simulink model "Accelerometer"  (R2020b)
settings: Solver=FixedStepDiscrete  StartTime=0.0  StopTime=10.0  FixedStep=0.01  RelTol=1e-3  EnableMultiTasking=on
InitFcn:
  | mbd_s32k_consistency_checks(bdroot(gcs));
undefined symbols (not defined in the file): LQFP
libraries: mbd_s32k1xx_ec_toolbox x18, simulink x10
Description:
  | Sample code for extracting X,Y,Z components of acceleration from the on-board sensor.
  | 
  | Extra Modules (In addition to template defaults):
  | LPSPI0 (Accelerometer connection)
  | 
  | For more information, see our Accelerometer Guide:
  | https://www.audesseinc.com/labs/resources/accelerometer-guide/
  | 
  | Revision: 1.2
settings Model: LastModifiedBy=prasa
settings DataIOCC: ExternalInput=off  InitialState=off  SaveOutput=off  SignalLogging=off  SaveTime=off
settings OptimizationCC: DefaultParameterBehavior=Inlined  DefaultUnderspecifiedDataType=single  EnhancedBackFolding=on  PassReuseOutputArgsAs=Individual arguments  OptimizeBlockOrder=speed  EfficientTunableParamExpr=on
settings DebuggingCC: InheritedTsInSrcMsg=none  SingleTaskRateTransMsg=error  ParameterTunabilityLossMsg=error  UnconnectedInputMsg=error  UnconnectedOutputMsg=error  UnconnectedLineMsg=error  UnknownTsInhSupMsg=error  ArithmeticOperatorsInVariantConditions=warning
settings HardwareCC: ProdBitPerPointer=32  ProdBitPerSizeT=32  ProdBitPerPtrDiffT=32  ProdLargestAtomicInteger=Long  ProdLargestAtomicFloat=Double  ProdWordSize=32  ProdHWDeviceType=ARM Compatible->ARM Cortex
settings SFSimCC: MATLABDynamicMemAlloc=off  CustomCodeUndefinedFunction=UseInterfaceOnly
settings RTWCC: Description=Model Based Design Toolbox S32K1xx Code Generation Target  SystemTargetFile=mbd_s32k.tlc  MakeCommand=mbd_s32k_make_rtw COPY_MDLREF_INCLUDES=0  TemplateMakefile=mbd_s32k.tmf  GenerateReport=on  IncludeHyperlinkInReport=on  LaunchReport=on  GenerateTraceInfo=on  GenerateTraceReport=on  GenerateTraceReportSl=on  GenerateTraceReportSf=on  GenerateTraceReportEml=on
settings CodeAppCC: ForceParamTrailComments=on  IgnoreCustomStorageClasses=off  OperatorAnnotations=on  SimulinkDataObjDesc=on  SFDataObjDesc=on  InsertBlockDesc=on  StateflowObjectComments=on
settings STFCustomTargetCC: TargetLangStandard=C99 (ISO)  MultiwordLength=256  ConcurrentExecutionCompliant=off  CombineOutputUpdateFcns=on  ERTCustomFileBanners=on  SupportContinuousTime=off  SupportNonInlinedSFcns=off  RemoveResetFunc=on  MATLABClassNameForMDSCustomization=Simulink.SoftwareTarget.ERTCustomization  CPPClassGenCompliant=off  GRTInterface=off  SystemTargetFile=mbd_s32k.tlc
settings ERTTargetCC: TargetLangStandard=C99 (ISO)  ParMdlRefBuildCompliant=off  CompOptLevelCompliant=off  ConcurrentExecutionCompliant=off  ModelStepFunctionPrototypeControlCompliant=off  CPPClassGenCompliant=off  UseToolchainInfoCompliant=off  InlinedParameterPlacement=NonHierarchical  ERTSrcFileBannerTemplate=mbd_ert_code_template.cgt  ERTHdrFileBannerTemplate=mbd_ert_code_template.cgt  ERTDataSrcFileTemplate=mbd_ert_code_template.cgt  ERTDataHdrFileTemplate=mbd_ert_code_template.cgt  ERTCustomFileTemplate=example_file_process.tlc

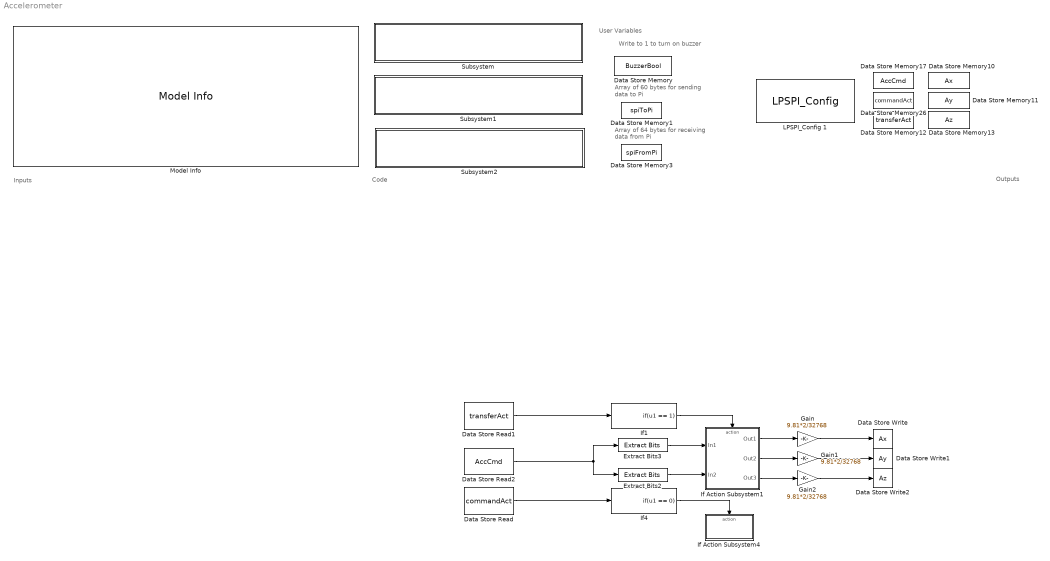
== system Accelerometer ==
  note: User Variables
  note: Write to 1 to turn on buzzer
  note: Array of 60 bytes for sending data to Pi
  note: Inputs
  note: Code
  note: Outputs
  note: Array of 64 bytes for receiving data from Pi
  Data Store Memory : DataStoreMemory  DataStoreName=BuzzerBool  ReadBeforeWriteMsg=warning  WriteAfterWriteMsg=warning  WriteAfterReadMsg=warning  ShowAdditionalParam=off  OutDataTypeStr=boolean
  Data Store Memory1 : DataStoreMemory  DataStoreName=spiToPi  ReadBeforeWriteMsg=warning  WriteAfterWriteMsg=warning  WriteAfterReadMsg=warning  InitialValue=255*ones(1,60)  ShowAdditionalParam=off  OutDataTypeStr=uint8
  Data Store Memory10 : DataStoreMemory  DataStoreName=Ax  ReadBeforeWriteMsg=warning  WriteAfterWriteMsg=warning  WriteAfterReadMsg=warning  InitialValue=[0]  ShowAdditionalParam=off  OutDataTypeStr=single
  Data Store Memory11 : DataStoreMemory  DataStoreName=Ay  ReadBeforeWriteMsg=warning  WriteAfterWriteMsg=warning  WriteAfterReadMsg=warning  InitialValue=[0]  ShowAdditionalParam=off  OutDataTypeStr=single
  Data Store Memory12 : DataStoreMemory  DataStoreName=transferAct  ReadBeforeWriteMsg=warning  WriteAfterWriteMsg=warning  WriteAfterReadMsg=warning  InitialValue=[1]  ShowAdditionalParam=off  OutDataTypeStr=boolean
  Data Store Memory13 : DataStoreMemory  DataStoreName=Az  ReadBeforeWriteMsg=warning  WriteAfterWriteMsg=warning  WriteAfterReadMsg=warning  InitialValue=[0]  ShowAdditionalParam=off  OutDataTypeStr=single
  Data Store Memory17 : DataStoreMemory  DataStoreName=AccCmd  ReadBeforeWriteMsg=warning  WriteAfterWriteMsg=warning  WriteAfterReadMsg=warning  InitialValue=[8208]  ShowAdditionalParam=off  OutDataTypeStr=uint16
  Data Store Memory26 : DataStoreMemory  DataStoreName=commandAct  ReadBeforeWriteMsg=warning  WriteAfterWriteMsg=warning  WriteAfterReadMsg=warning  InitialValue=[0]  ShowAdditionalParam=off  OutDataTypeStr=boolean
  Data Store Memory3 : DataStoreMemory  DataStoreName=spiFromPi  ReadBeforeWriteMsg=warning  WriteAfterWriteMsg=warning  WriteAfterReadMsg=warning  InitialValue=zeros(1,64)  ShowAdditionalParam=off  OutDataTypeStr=uint8
  Data Store Read : DataStoreRead  DataStoreName=commandAct
  Data Store Read1 : DataStoreRead  DataStoreName=transferAct
  Data Store Read2 : DataStoreRead  DataStoreName=AccCmd
  Data Store Write : DataStoreWrite  DataStoreName=Ax
  Data Store Write1 : DataStoreWrite  DataStoreName=Ay
  Data Store Write2 : DataStoreWrite  DataStoreName=Az
  Extract Bits2 : simulink/Logic and Bit Operations/Extract Bits  bitsToExtract=Lower half  numBits=8  bitIdxRange=[0 7]  outScalingMode=Treat bit field as an integer
  Extract Bits3 : simulink/Logic and Bit Operations/Extract Bits  bitsToExtract=Upper half  numBits=8  bitIdxRange=[0 7]  outScalingMode=Treat bit field as an integer
  Gain : Gain  Gain=9.81*2/32768  OutDataTypeStr=single
  Gain1 : Gain  Gain=9.81*2/32768  OutDataTypeStr=single
  Gain2 : Gain  Gain=9.81*2/32768  OutDataTypeStr=single
  If Action Subsystem1 : Subsystem  TreatAsAtomicUnit=on
  If Action Subsystem4 : Subsystem  TreatAsAtomicUnit=on
  If1 : If  IfExpression=u1 == 1  ShowElse=off
  If4 : If  IfExpression=u1 == 0  ShowElse=off
  LPSPI_Config 1 : mbd_s32k1xx_ec_toolbox/Communication Blocks/SPI Blocks/LPSPI_Config   Priority=0  InstanceNumber=0  Role=Master  BaudRate=5000000  ShowAdvanced=on  sin=PTE1: [LPSPI0_SIN | LPSPI Serial Data Input]  sout=PTE2: [LPSPI0_SOUT | LPSPI Serial Data Output]  sck=PTE0: [LPSPI0_SCK | LPSPI Serial Clock I/O]  pcs0=None  pcs1=None  pcs2=None  pcs3=None  CPHA=1  CPOL=1  BitOrder=MSB first  TransferSize=8  WhichPCS=0  PCSPol=ActiveLow  ContinuousTransfer=on
  Model Info : simulink/Model-Wide Utilities/Model Info  Frame=on  DisplayStringWithTags=|  HorizontalTextAlignment=Left  LeftAlignmentValue=0.02
      | Audesse Simulink Samples: %<ModelName>
      | 
      | %<Description>
  Subsystem : Subsystem  Priority=1
      mask Display:
      | scl=1/4;
      | patch(scl*[0,52,90,54],scl*[16,55,146,146],[16/255,118/255,188/255],'bottom-left');
      | patch(scl*[0,27,82,77,68],scl*[16,0,42,62,69],[46/255,49/255,146/255],'bottom-left');
      | patch(scl*[89,125,90,68],scl*[16,16,146,91],[0,0,0],'bottom-left');
      | disp('Hardware Modules Config\n(SPI,CAN,ADC,etc..)');
  Subsystem1 : Subsystem
      mask Display:
      | scl=1/4;
      | patch(scl*[0,52,90,54],scl*[16,55,146,146],[16/255,118/255,188/255],'bottom-left');
      | patch(scl*[0,27,82,77,68],scl*[16,0,42,62,69],[46/255,49/255,146/255],'bottom-left');
      | patch(scl*[89,125,90,68],scl*[16,16,146,91],[0,0,0],'bottom-left');
      | disp('Default Control Functions\n(Do not modify unless you know what you are doing)');
  Subsystem2 : Subsystem
      mask Display:
      | scl=1/4;
      | patch(scl*[0,52,90,54],scl*[16,55,146,146],[16/255,118/255,188/255],'bottom-left');
      | patch(scl*[0,27,82,77,68],scl*[16,0,42,62,69],[46/255,49/255,146/255],'bottom-left');
      | patch(scl*[89,125,90,68],scl*[16,16,146,91],[0,0,0],'bottom-left');
      | disp('Run Once at Startup');
  wires:
  If Action Subsystem1/1(Out1) -> Gain/1
  Gain1/1 -> Data Store Write1/1
  Gain/1 -> Data Store Write/1
  If Action Subsystem1/3(Out3) -> Gain2/1
  Extract Bits2/1 -> If Action Subsystem1/2(In2)
  If Action Subsystem1/2(Out2) -> Gain1/1
  Gain2/1 -> Data Store Write2/1
  If1/1 -> If Action Subsystem1/Action
  Extract Bits3/1 -> If Action Subsystem1/1(In1)
  Data Store Read1/1 -> If1/1
  Data Store Read2/1 -> Extract Bits2/1, Extract Bits3/1
  If4/1 -> If Action Subsystem4/Action
  Data Store Read/1 -> If4/1

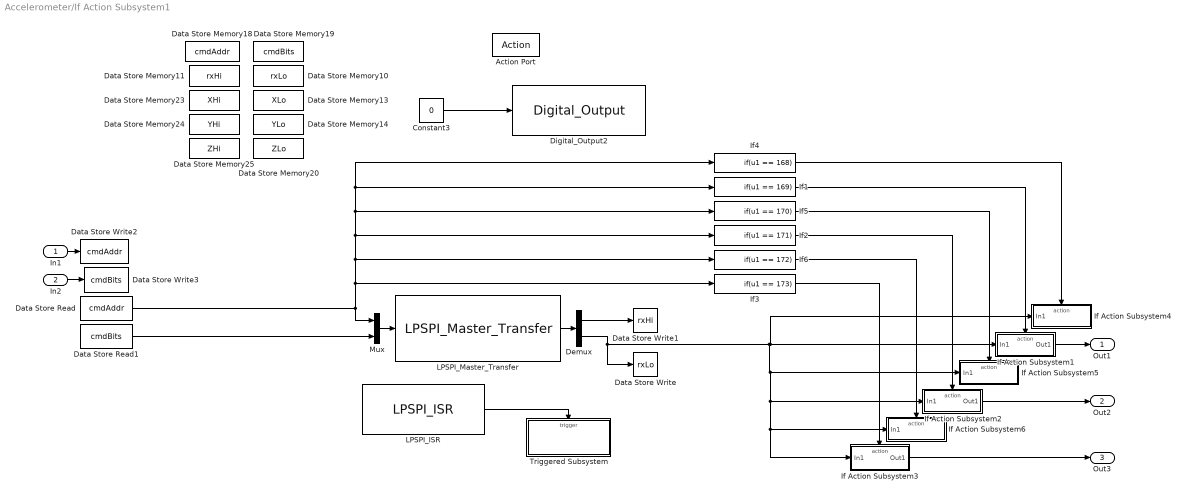
== system Accelerometer/If Action Subsystem1 ==
  In1 : Inport
  In2 : Inport  Port=2
  Action Port : ActionPort  ActionPortLabel=if(u1 == 1)
  Constant3 : Constant  Value=0  OutDataTypeStr=boolean
  Data Store Memory10 : DataStoreMemory  DataStoreName=rxLo  ReadBeforeWriteMsg=warning  WriteAfterWriteMsg=warning  WriteAfterReadMsg=warning  InitialValue=[0]  ShowAdditionalParam=off  OutDataTypeStr=uint8
  Data Store Memory11 : DataStoreMemory  DataStoreName=rxHi  ReadBeforeWriteMsg=warning  WriteAfterWriteMsg=warning  WriteAfterReadMsg=warning  InitialValue=[0]  ShowAdditionalParam=off  OutDataTypeStr=uint8
  Data Store Memory13 : DataStoreMemory  DataStoreName=XLo  ReadBeforeWriteMsg=warning  WriteAfterWriteMsg=warning  WriteAfterReadMsg=warning  InitialValue=[255]  ShowAdditionalParam=off  OutDataTypeStr=uint8
  Data Store Memory14 : DataStoreMemory  DataStoreName=YLo  ReadBeforeWriteMsg=warning  WriteAfterWriteMsg=warning  WriteAfterReadMsg=warning  InitialValue=[255]  ShowAdditionalParam=off  OutDataTypeStr=uint8
  Data Store Memory18 : DataStoreMemory  DataStoreName=cmdAddr  ReadBeforeWriteMsg=warning  WriteAfterWriteMsg=warning  WriteAfterReadMsg=warning  InitialValue=[0]  ShowAdditionalParam=off  OutDataTypeStr=uint8
  Data Store Memory19 : DataStoreMemory  DataStoreName=cmdBits  ReadBeforeWriteMsg=warning  WriteAfterWriteMsg=warning  WriteAfterReadMsg=warning  InitialValue=[0]  ShowAdditionalParam=off  OutDataTypeStr=uint8
  Data Store Memory20 : DataStoreMemory  DataStoreName=ZLo  ReadBeforeWriteMsg=warning  WriteAfterWriteMsg=warning  WriteAfterReadMsg=warning  InitialValue=[255]  ShowAdditionalParam=off  OutDataTypeStr=uint8
  Data Store Memory23 : DataStoreMemory  DataStoreName=XHi  ReadBeforeWriteMsg=warning  WriteAfterWriteMsg=warning  WriteAfterReadMsg=warning  InitialValue=[255]  ShowAdditionalParam=off  OutDataTypeStr=uint8
  Data Store Memory24 : DataStoreMemory  DataStoreName=YHi  ReadBeforeWriteMsg=warning  WriteAfterWriteMsg=warning  WriteAfterReadMsg=warning  InitialValue=[255]  ShowAdditionalParam=off  OutDataTypeStr=uint8
  Data Store Memory25 : DataStoreMemory  DataStoreName=ZHi  ReadBeforeWriteMsg=warning  WriteAfterWriteMsg=warning  WriteAfterReadMsg=warning  InitialValue=[255]  ShowAdditionalParam=off  OutDataTypeStr=uint8
  Data Store Read : DataStoreRead  Priority=2  DataStoreName=cmdAddr
  Data Store Read1 : DataStoreRead  Priority=3  DataStoreName=cmdBits
  Data Store Write : DataStoreWrite  DataStoreName=rxLo
  Data Store Write1 : DataStoreWrite  DataStoreName=rxHi
  Data Store Write2 : DataStoreWrite  Priority=2  DataStoreName=cmdAddr
  Data Store Write3 : DataStoreWrite  Priority=3  DataStoreName=cmdBits
  Demux : Demux  Outputs=2
  Digital_Output2 : mbd_s32k1xx_ec_toolbox/GPIO Blocks/Digital_Output  Priority=1  gpio_pin=PTA11: [PTA11 | Port A I/O]  init_val=High  drive_strength=Low
  If Action Subsystem1 : Subsystem  TreatAsAtomicUnit=on
  If Action Subsystem2 : Subsystem  TreatAsAtomicUnit=on
  If Action Subsystem3 : Subsystem  TreatAsAtomicUnit=on
  If Action Subsystem4 : Subsystem  TreatAsAtomicUnit=on
  If Action Subsystem5 : Subsystem  TreatAsAtomicUnit=on
  If Action Subsystem6 : Subsystem  TreatAsAtomicUnit=on
  If1 : If  IfExpression=u1 == 169  ShowElse=off
  If2 : If  IfExpression=u1 == 171  ShowElse=off
  If3 : If  IfExpression=u1 == 173  ShowElse=off
  If4 : If  IfExpression=u1 == 168  ShowElse=off
  If5 : If  IfExpression=u1 == 170  ShowElse=off
  If6 : If  IfExpression=u1 == 172  ShowElse=off
  LPSPI_ISR : mbd_s32k1xx_ec_toolbox/Communication Blocks/SPI Blocks/LPSPI_ISR  instanceNumber=0  isr_lvl=0  role=Master  transfer_end=on  spi_upd=on
  LPSPI_Master_Transfer : mbd_s32k1xx_ec_toolbox/Communication Blocks/SPI Blocks/LPSPI_Master_Transfer  Priority=15  instance=0  pcs=0  pcs_polarity=ActiveLow  xfermode=Non blocking  timeout=50  spi_upd=on
  Mux : Mux  Inputs=2
  Triggered Subsystem : Subsystem  TreatAsAtomicUnit=on
  Out1 : Outport  VectorParamsAs1DForOutWhenUnconnected=off
  Out2 : Outport  Port=2  VectorParamsAs1DForOutWhenUnconnected=off
  Out3 : Outport  Port=3  VectorParamsAs1DForOutWhenUnconnected=off
  wires:
  LPSPI_Master_Transfer/1 -> Demux/1
  Demux/1 -> Data Store Write1/1
  LPSPI_ISR/1 -> Triggered Subsystem/Trigger
  Mux/1 -> LPSPI_Master_Transfer/1
  Constant3/1 -> Digital_Output2/1
  If1/1 -> If Action Subsystem1/Action
  If2/1 -> If Action Subsystem2/Action
  If3/1 -> If Action Subsystem3/Action
  If4/1 -> If Action Subsystem4/Action
  If5/1 -> If Action Subsystem5/Action
  If6/1 -> If Action Subsystem6/Action
  Demux/2 -> If Action Subsystem4/1(In1), If Action Subsystem1/1(In1), If Action Subsystem3/1(In1), If Action Subsystem6/1(In1), If Action Subsystem2/1(In1), If Action Subsystem5/1(In1), Data Store Write/1
  In1/1 -> Data Store Write2/1
  In2/1 -> Data Store Write3/1
  Data Store Read/1 -> Mux/1, If3/1, If6/1, If2/1, If4/1, If1/1, If5/1
  Data Store Read1/1 -> Mux/2
  If Action Subsystem1/1(Out1) -> Out1/1
  If Action Subsystem2/1(Out1) -> Out2/1
  If Action Subsystem3/1(Out1) -> Out3/1

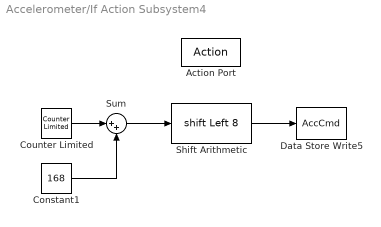
== system Accelerometer/If Action Subsystem4 ==
  Action Port : ActionPort  ActionPortLabel=if(u1 == 0)
  Constant1 : Constant  Value=168  OutDataTypeStr=uint16
  Counter Limited : simulink/Sources/Counter Limited  uplimit=5  tsamp=-1
  Data Store Write5 : DataStoreWrite  DataStoreName=AccCmd
  Shift Arithmetic : ArithShift  BitShiftNumber=8  BitShiftDirection=Left
  Sum : Sum  Inputs=|++
  wires:
  Shift Arithmetic/1 -> Data Store Write5/1
  Sum/1 -> Shift Arithmetic/1
  Counter Limited/1 -> Sum/1
  Constant1/1 -> Sum/2

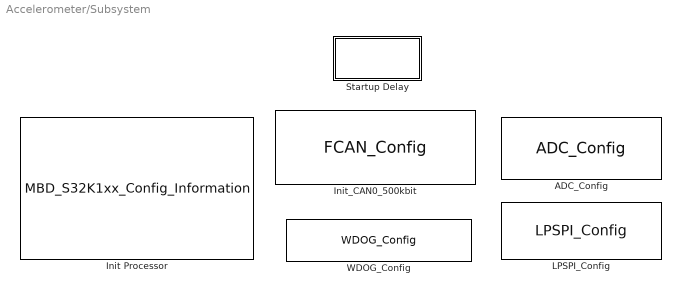
== system Accelerometer/Subsystem ==
  ADC_Config : mbd_s32k1xx_ec_toolbox/Motor Control Blocks/ADC Blocks/ADC_Config  instance=0  mode=12-bit conversion  smplts=20  adiclk=alternate clock 1  adiv=input clock  show_adv_opts=on  pretrgsel=PDB pre-trigger  swpretrg=Disabled  adtrg=software  trgsel=TRGMUX output  refsel=Vrefh and Vrefl  supply_monitoring=off  acfe=off  acfgt=off  acren=off  cv1=0  cv2=0  adco=off  avge=off  avgs=4 samples
  Init Processor : mbd_s32k1xx_ec_toolbox/MBD_S32K1xx_Config_Information  mbdt_ver=0  disp_str=|  config_params=[]  mcu_target_name=S32K144  mcu_target_package=100-LQFP  mcu_target_sram_size=64KB  mcu_system_clock_freq=80  mcu_xtal_freq=External 8  mcu_steptick_timer=LPIT Channel 0  mcu_steptick_prio=15  ds_import_enable=on  target_compiler=GCC  target_memory=FLASH  gcc_target_compile_opts=-mcpu=cortex-m4 -mthumb -mfloat-abi=hard -mfpu=fpv4-sp-d16 -O1 -g -gstrict-dwarf  gcc_target_assemble_opts=-mcpu=cortex-m4 -mthumb -mfloat-abi=hard -mfpu=fpv4-sp-d16 -g  gcc_target_link_opts=-mcpu=cortex-m4 -mthumb -mfloat-abi=hard -mfpu=fpv4-sp-d16  gcc_target_default_lcf=on  gcc_target_user_lcf=S32K148_192_flash.ld  ghs_target_compile_opts=-cpu=cortexm4f -thumb -DARM_MATH_CM4 -fpu=vfpv4_d16 -fsingle -Ogeneral -Wundef -Wimplicit-int -Wshadow -Wtrigraphs --no_commons --gnu_asm -gnu99 -gdwarf-2 -G  ghs_target_assemble_opts=-cpu=cortexm4f -fpu=vfpv4_d16  ghs_target_link_opts=-cpu=cortexm4f -thumb -fpu=vfpv4_d16  ghs_target_default_lcf=on  ghs_target_user_lcf=S32K148_192_flash.ld  iar_target_compile_opts=--cpu=Cortex-M4F --thumb --fpu=VFPv4_sp -Ol -e --debug --dlib_config normal  iar_target_assemble_opts=--cpu Cortex-M4F --thumb --fpu VFPv4_sp  iar_target_link_opts=--no_exceptions --vfe --inline  iar_target_default_lcf=on  iar_target_user_lcf=S32K148_192_flash.icf  pil_download_enable=off  rbl_download_enable=off  rbl_start_delay=5000000  rbl_download_interface=OpenSDA  rbl_restart_request=off  rbl_com_port=Custom  rbl_com_port_custom=COM1  pil_download_rate=57600  pil_opensda_drive=Custom  pil_opensda_drive_custom=D  pil_uart_instance=1  pil_uart_rx=PTC6: [LPUART1_RX | Receive]  pil_uart_tx=PTC7: [LPUART1_TX | Transmit]  FTM_PWM_PcrCheckEnDis=on  FTM_Input_Edge_Inputs_PcrCheckEnDis=on  FTM_Dual_Edge_Inputs_PcrCheckEnDis=on  FTM_Quadrature_Inputs_PcrCheckEnDis=on  FTM_Hall_Sensor_Inputs_PcrCheckEnDis=on  LPTMR_PcrCheckEnDis=on  PIT_PcrCheckEnDis=on  RTC_PcrCheckEnDis=on  FlexCAN_PcrCheckEnDis=on  LIN_PcrCheckEnDis=on  FlexIO_PcrCheckEnDis=on  LPI2C_PcrCheckEnDis=on  LPSPI_PcrCheckEnDis=on  LPUART_PcrCheckEnDis=on  CMP_PcrCheckEnDis=on  GPIO_OutputPcrCheckEnDis=on  GPIO_InputPcrCheckEnDis=on  SBC_PcrCheckEnDis=on  BMS_PcrCheckEnDis=on  AMMCLIB_PcrCheckEnDis=on  FM_PcrCheckEnDis=on  Profile_PcrCheckEnDis=on  ConfigParams_PcrCheckEnDis=on  ModelRef_PcrCheckEnDis=on  PDB0_PcrCheckEnDis=on  CSEc_PcrCheckEnDis=on  eDMA_PcrCheckEnDis=on  FLASH_PcrCheckEnDis=on  ADC_PcrCheckEnDis=on  WDOG_PcrCheckEnDis=on
      | Target : S32K144-64KB_SRAM
      | Package : 100-pin
      | System clock : 80 MHz
      | XTAL clock : External 8 MHz
      | Compiler : IAR
      | Target Type : FLASH
      | Download Code after build : off
      | Step Tick Interrupt Priority : 15
  Init_CAN0_500kbit : mbd_s32k1xx_ec_toolbox/Communication Blocks/CAN Blocks/FCAN_Config  can_instance=0  can_mode=Normal mode  can_max_num_mb=16  can_rx=PTB0: [CAN0_RX | CAN Rx channel]  can_tx=PTB1: [CAN0_TX | CAN Tx Channel]  show_adv_opts=off  can_clk_src=Peripheral clock  bitrate=500  bitrate_adv_opts=off  can_presdiv=7  can_rjw=3  can_pseg1=6  can_pseg2=3  can_propseg=7  can_cbt_presdiv=9  can_cbt_rjw=0  can_cbt_pseg1=3  can_cbt_pseg2=3  can_cbt_propseg=6  can_fd_enable=off  can_payload=8  can_rxfifo_enable=off  can_fifo_id_filter_extended=off  can_fifo_id_filter_remote=off  can_num_id_filters=8  can_fifo_id_format=A  can_fifo_id_filter={'0x0', '0x0', '0x0', '0x0', '0x0', '0x0', '0x0', '0x0'}  can_pn_enable=off  can_wakeup_match=off  can_wakeup_timeout=off  can_timeout_en=off  can_match_timeout=1  can_multiple_matches_en=off  can_num_matches=1  can_idfilter_extendedid=off  can_idfilter_remoteframe=off  can_idfilter_type=Match exact  can_idfilter_id1=0  can_idfilter_id2=0  can_payloadfilter_enable=on  can_payloadfilter_dlclow=0  can_payloadfilter_dlchigh=0  can_payloadfilter_type=Match exact  can_payloadfilter_payload1_b0=0  can_payloadfilter_payload1_b1=0  can_payloadfilter_payload1_b2=0  can_payloadfilter_payload1_b3=0  can_payloadfilter_payload1_b4=0  can_payloadfilter_payload1_b5=0  can_payloadfilter_payload1_b6=0  can_payloadfilter_payload1_b7=0  can_payloadfilter_payload2_b0=0  can_payloadfilter_payload2_b1=0  can_payloadfilter_payload2_b2=0  can_payloadfilter_payload2_b3=0  can_payloadfilter_payload2_b4=0  can_payloadfilter_payload2_b5=0  can_payloadfilter_payload2_b6=0  can_payloadfilter_payload2_b7=0
  "LPSPI_Config " : mbd_s32k1xx_ec_toolbox/Communication Blocks/SPI Blocks/LPSPI_Config   InstanceNumber=1  Role=Slave  BaudRate=10000  ShowAdvanced=on  sin=PTB15: [LPSPI1_SIN | LPSPI Serial Data Input]  sout=PTB16: [LPSPI1_SOUT | LPSPI Serial Data Output]  sck=PTB14: [LPSPI1_SCK | LPSPI Serial Clock I/O]  pcs0=None  pcs1=None  pcs2=None  pcs3=PTB17: [LPSPI1_PCS3 | Peripheral Chip Select 3]  CPHA=1  CPOL=0  BitOrder=MSB first  TransferSize=8  WhichPCS=0  PCSPol=ActiveLow  ContinuousTransfer=on
  Startup Delay : Subsystem  mask(System Start){ShowInLibBrowser=0}
      mask prompts: ShowInLibBrowser "Simulink:masks:CustCodeMaskParam1_MP"
      settings: CopyFcn=cccopyfcn(gcb)  OpenFcn=ccopenfcn('System Start Function')
      mask Help: eval('feval(''rtwprivate'',''rtwhelpview'',''rtw_sys_start_block'')');
      mask Display: disp('System\nStart');
  WDOG_Config : mbd_s32k1xx_ec_toolbox/Core and System Blocks/WDOG Blocks/WDOG_Config  clk_source=LPO clock  window_enable=off  window_value=1000.000 milliseconds  timeout_value=1000.000 milliseconds  prescaler_enable=on  update_enable=off  int_enable=off  show_adv_opts=on

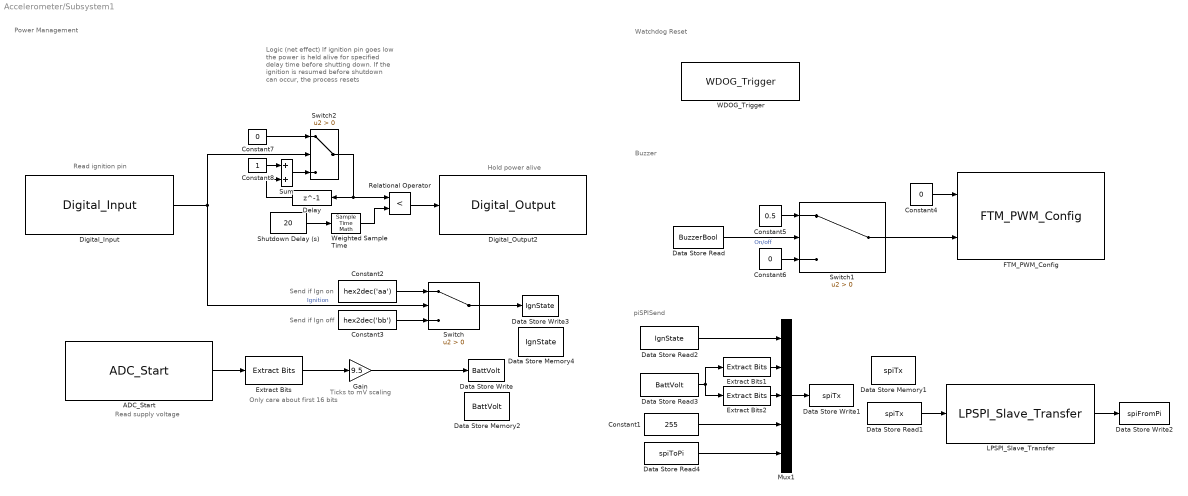
== system Accelerometer/Subsystem1 ==
  note: piSPISend
  note: Watchdog Reset
  note: Power Management
  note: Read ignition pin
  note: Only care about
      | first 16 bits
  note: Ticks to mV scaling
  note: Read supply voltage
  note: Send if Ign on
  note: Send if Ign off
  note: Buzzer
  note: Logic (net effect)
      | If ignition pin goes low the power is held alive for specified delay time before shutting down.
      |
      | If the ignition is resumed before shutdown can occur, the process resets
  note: Hold power alive
  ADC_Start : mbd_s32k1xx_ec_toolbox/Motor Control Blocks/ADC Blocks/ADC_Start  instance=0  adc_r=A  adc_chan=PTA6: [ADC0_SE2 | ADC Single Ended Input]  aien=off  mcuTargetUpdate=on
  Constant1 : Constant  Value=255  OutDataTypeStr=uint8
  Constant2 : Constant  Value=hex2dec('aa')  OutDataTypeStr=uint8
  Constant3 : Constant  Value=hex2dec('bb')  OutDataTypeStr=uint8
  Constant4 : Constant  Value=0  OutDataTypeStr=single
  Constant5 : Constant  Value=0.5  OutDataTypeStr=single
  Constant6 : Constant  Value=0  OutDataTypeStr=single
  Constant7 : Constant  Value=0  OutDataTypeStr=uint8
  Constant8 : Constant  OutDataTypeStr=uint8
  Data Store Memory1 : DataStoreMemory  DataStoreName=spiTx  ReadBeforeWriteMsg=warning  WriteAfterWriteMsg=warning  WriteAfterReadMsg=warning  InitialValue=zeros(1,64)  ShowAdditionalParam=off  OutDataTypeStr=uint8
  Data Store Memory2 : DataStoreMemory  DataStoreName=BattVolt  ReadBeforeWriteMsg=warning  WriteAfterWriteMsg=warning  WriteAfterReadMsg=warning  InitialValue=[0]  ShowAdditionalParam=off  OutDataTypeStr=uint16
  Data Store Memory4 : DataStoreMemory  DataStoreName=IgnState  ReadBeforeWriteMsg=warning  WriteAfterWriteMsg=warning  WriteAfterReadMsg=warning  InitialValue=[170]  ShowAdditionalParam=off  OutDataTypeStr=uint8
  Data Store Read : DataStoreRead  DataStoreName=BuzzerBool
  Data Store Read1 : DataStoreRead  DataStoreName=spiTx
  Data Store Read2 : DataStoreRead  DataStoreName=IgnState
  Data Store Read3 : DataStoreRead  DataStoreName=BattVolt
  Data Store Read4 : DataStoreRead  DataStoreName=spiToPi
  Data Store Write : DataStoreWrite  DataStoreName=BattVolt
  Data Store Write1 : DataStoreWrite  DataStoreName=spiTx
  Data Store Write2 : DataStoreWrite  DataStoreName=spiFromPi
  Data Store Write3 : DataStoreWrite  DataStoreName=IgnState
  Delay : Delay  DelayLength=1  InitialCondition=0
  Digital_Input : mbd_s32k1xx_ec_toolbox/GPIO Blocks/Digital_Input  gpio_pin=PTE13: [PTE13 | Port E I/O]  pull_resistor=Pulldown  passive_filter=off
  Digital_Output2 : mbd_s32k1xx_ec_toolbox/GPIO Blocks/Digital_Output  gpio_pin=PTD7: [PTD7 | Port D I/O]  init_val=High  drive_strength=Low
  Extract Bits : simulink/Logic and Bit Operations/Extract Bits  bitsToExtract=Lower half  numBits=8  bitIdxRange=[0 7]  outScalingMode=Treat bit field as an integer
  Extract Bits1 : simulink/Logic and Bit Operations/Extract Bits  bitsToExtract=Upper half  numBits=8  bitIdxRange=[0 7]  outScalingMode=Treat bit field as an integer
  Extract Bits2 : simulink/Logic and Bit Operations/Extract Bits  bitsToExtract=Lower half  numBits=8  bitIdxRange=[0 7]  outScalingMode=Treat bit field as an integer
  FTM_PWM_Config : mbd_s32k1xx_ec_toolbox/Motor Control Blocks/FTM Blocks/FTM_PWM_Config  ftmModule=2  ftmMode=Edge-Aligned PWM  ftmSourceClock=80 MHz  swcontrol_enable=off  chan0En=off  chan0Type=Complementary  chan2En=on  chan2Type=Independent  chan4En=off  chan4Type=Independent  chan6En=off  chan6Type=Independent  ftmPwmUnits=Hz  outFrequency=4000  ftmPeriod=20000  ftmPrescaler=Divide by 1  deadtimeUnits=Nanoseconds  deadtimeNs=0  deadtimeTicks=0  deadtimePrescaler=Divide by 1  dutyCycleCh0=0.25  dutyCycleCh1=0.25  dutyCycleCh2=0  dutyCycleCh3=0.5  dutyCycleCh4=0.25  dutyCycleCh5=0.25  dutyCycleCh6=0.25  dutyCycleCh7=0.25  dutyCycleSim=off  startAfterInit=on  showAdvOpt=on  pinFtmCh0=PTC5: [FTM2_CH0 | FTM Channel]  pinFtmCh1=None  pinPolCh0=Active Low  pinPolCh1=Active Low  outputComplem0=Main duplicated  outputLevel0=Low  outputLevel1=Low  pinFtmCh2=PTE4: [FTM2_CH2 | FTM Channel]  pinFtmCh3=PTD5: [FTM2_CH3 | FTM Channel]  pinPolCh2=Active Low  pinPolCh3=Active High  outputComplem2=Main duplicated  outputLevel2=High  outputLevel3=Low  pinFtmCh4=PTD13: [FTM2_CH4 | FTM Channel]  pinFtmCh5=None  pinPolCh4=Active Low  pinPolCh5=Active Low  outputComplem4=Main duplicated  outputLevel4=Low  outputLevel5=Low  pinFtmCh6=PTC12: [FTM2_CH6 | FTM Channel]  pinFtmCh7=None  pinPolCh6=Active Low  pinPolCh7=Active Low  outputComplem6=Main duplicated  outputLevel6=Low  outputLevel7=Low  initTrigger=off  chTrigger0=off  chTrigger1=off  chTrigger2=off  chTrigger3=off  chTrigger4=off  chTrigger5=off  chTrigger6=off  chTrigger7=off  mcuTargetUpdate=on  pwmSyncTrg=Software trigger  pwmSyncHwRouting=TRGMUX_FTM7  pwmSyncTrg0=off  pwmSyncTrg1=off  pwmSyncTrg2=off  pwmSyncAutoClear=on  pwmSyncMinLoad=on  pwmSyncMaxLoad=on  pwmSyncInvert=System Clock  pwmSyncOutControl=System Clock  pwmSyncOutMask=System Clock  pwmSyncCounterInitial=System Clock  pwmSyncPoints=Update now  reloadEnable=off  reloadPriority=15  reloadHalfCycle=off  reloadHCR=0  reloadFrequency=0  chnMatch0=off  chnMatch1=off  chnMatch2=off  chnMatch3=off  chnMatch4=off  chnMatch5=off  chnMatch6=off  chnMatch7=off  pwmFaultProtection=off  pwmFaultInterrupt=off  pwmFaultClearing=Fault control disabled  pwmFaultPinState=Safe Value  pwmFaultFilterValue=0  pwmFaultPriority=15  fault_disen_0=off  fault_filter_0=off  fault_polarity_0=Active High  fault_disen_1=off  fault_filter_1=off  fault_polarity_1=Active high  fault_disen_2=off  fault_filter_2=off  fault_polarity_2=Active high  fault_disen_3=off  fault_filter_3=off  fault_polarity_3=Active high  fault_pin_0=None  fault_pin_1=None  fault_pin_2=None  fault_pin_3=None
  Gain : Gain  Gain=9.5  OutDataTypeStr=uint16
  LPSPI_Slave_Transfer : mbd_s32k1xx_ec_toolbox/Communication Blocks/SPI Blocks/LPSPI_Slave_Transfer  instance=1  pcs=3  pcs_polarity=ActiveLow  xfermode=Non blocking  timeout=70  spi_upd=on
  Mux1 : Mux  Inputs=5
  Relational Operator : RelationalOperator  Operator=<  OutDataTypeStr=boolean  RndMeth=Simplest  InputSameDT=on
  Shutdown Delay (s) : Constant  Value=20  OutDataTypeStr=uint32
  Sum : Sum
  Switch : Switch  Criteria=u2 > Threshold
  Switch1 : Switch  Criteria=u2 > Threshold  OutDataTypeStr=single
  Switch2 : Switch  Criteria=u2 > Threshold  OutDataTypeStr=uint32
  WDOG_Trigger : mbd_s32k1xx_ec_toolbox/Core and System Blocks/WDOG Blocks/WDOG_Trigger
  Weighted Sample Time : SampleTimeMath  TsampMathOp=/  OutDataTypeStr=Inherit: Inherit via back propagation  RndMeth=Round  SaturateOnIntegerOverflow=on
  wires:
  Constant3/1 -> Switch/3
  Constant2/1 -> Switch/1
  Extract Bits/1 -> Gain/1
  ADC_Start/1 -> Extract Bits/1
  Switch/1 -> Data Store Write3/1
  Data Store Read/1 -> Switch1/2  "On/off"
  Switch1/1 -> FTM_PWM_Config/2
  Constant5/1 -> Switch1/1
  Constant4/1 -> FTM_PWM_Config/1
  Constant6/1 -> Switch1/3
  Data Store Read2/1 -> Mux1/1
  Mux1/1 -> Data Store Write1/1
  Data Store Read1/1 -> LPSPI_Slave_Transfer/1
  LPSPI_Slave_Transfer/1 -> Data Store Write2/1
  Gain/1 -> Data Store Write/1
  Constant1/1 -> Mux1/4
  Data Store Read4/1 -> Mux1/5
  Extract Bits2/1 -> Mux1/3
  Extract Bits1/1 -> Mux1/2
  Data Store Read3/1 -> Extract Bits2/1, Extract Bits1/1
  Relational Operator/1 -> Digital_Output2/1
  Shutdown Delay (s)/1 -> Weighted Sample Time/1
  Weighted Sample Time/1 -> Relational Operator/2
  Switch2/1 -> Delay/1, Relational Operator/1
  Constant8/1 -> Sum/1
  Constant7/1 -> Switch2/1
  Digital_Input/1 -> Switch2/2, Switch/2  "Ignition"
  Sum/1 -> Switch2/3
  Delay/1 -> Sum/2

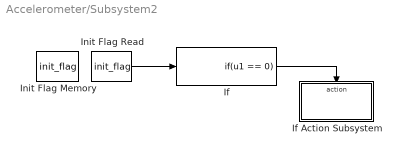
== system Accelerometer/Subsystem2 ==
  If : If  IfExpression=u1 == 0  ShowElse=off
  If Action Subsystem : Subsystem  TreatAsAtomicUnit=on
  Init Flag Memory : DataStoreMemory  DataStoreName=init_flag  ReadBeforeWriteMsg=warning  WriteAfterWriteMsg=warning  WriteAfterReadMsg=warning  ShowAdditionalParam=off  OutDataTypeStr=uint32
  Init Flag Read : DataStoreRead  DataStoreName=init_flag
  wires:
  Init Flag Read/1 -> If/1
  If/1 -> If Action Subsystem/Action

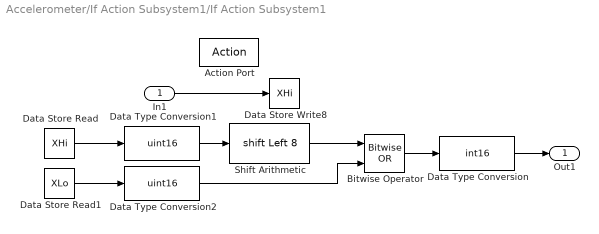
== system Accelerometer/If Action Subsystem1/If Action Subsystem1 ==
  In1 : Inport
  Action Port : ActionPort  ActionPortLabel=if(u1 == 169)
  Bitwise Operator : simulink/Logic and Bit Operations/Bitwise Operator  logicop=OR  UseBitMask=off  NumInputPorts=2  BitMask=bin2dec('11011001')  BitMaskRealWorld=Stored Integer
  Data Store Read : DataStoreRead  DataStoreName=XHi
  Data Store Read1 : DataStoreRead  DataStoreName=XLo
  Data Store Write8 : DataStoreWrite  DataStoreName=XHi
  Data Type Conversion : DataTypeConversion  OutDataTypeStr=int16
  Data Type Conversion1 : DataTypeConversion  OutDataTypeStr=uint16
  Data Type Conversion2 : DataTypeConversion  OutDataTypeStr=uint16
  Shift Arithmetic : ArithShift  BitShiftNumber=8  BitShiftDirection=Left
  Out1 : Outport  VectorParamsAs1DForOutWhenUnconnected=off
  wires:
  In1/1 -> Data Store Write8/1
  Data Store Read/1 -> Data Type Conversion1/1
  Data Store Read1/1 -> Data Type Conversion2/1
  Shift Arithmetic/1 -> Bitwise Operator/1
  Bitwise Operator/1 -> Data Type Conversion/1
  Data Type Conversion/1 -> Out1/1
  Data Type Conversion1/1 -> Shift Arithmetic/1
  Data Type Conversion2/1 -> Bitwise Operator/2

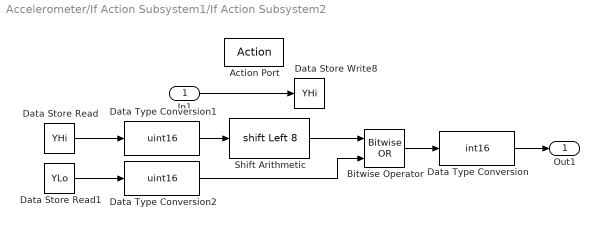
== system Accelerometer/If Action Subsystem1/If Action Subsystem2 ==
  In1 : Inport
  Action Port : ActionPort  ActionPortLabel=if(u1 == 171)
  Bitwise Operator : simulink/Logic and Bit Operations/Bitwise Operator  logicop=OR  UseBitMask=off  NumInputPorts=2  BitMask=bin2dec('11011001')  BitMaskRealWorld=Stored Integer
  Data Store Read : DataStoreRead  DataStoreName=YHi
  Data Store Read1 : DataStoreRead  DataStoreName=YLo
  Data Store Write8 : DataStoreWrite  DataStoreName=YHi
  Data Type Conversion : DataTypeConversion  OutDataTypeStr=int16
  Data Type Conversion1 : DataTypeConversion  OutDataTypeStr=uint16
  Data Type Conversion2 : DataTypeConversion  OutDataTypeStr=uint16
  Shift Arithmetic : ArithShift  BitShiftNumber=8  BitShiftDirection=Left
  Out1 : Outport  VectorParamsAs1DForOutWhenUnconnected=off
  wires:
  In1/1 -> Data Store Write8/1
  Data Store Read1/1 -> Data Type Conversion2/1
  Data Store Read/1 -> Data Type Conversion1/1
  Data Type Conversion/1 -> Out1/1
  Bitwise Operator/1 -> Data Type Conversion/1
  Data Type Conversion2/1 -> Bitwise Operator/2
  Shift Arithmetic/1 -> Bitwise Operator/1
  Data Type Conversion1/1 -> Shift Arithmetic/1

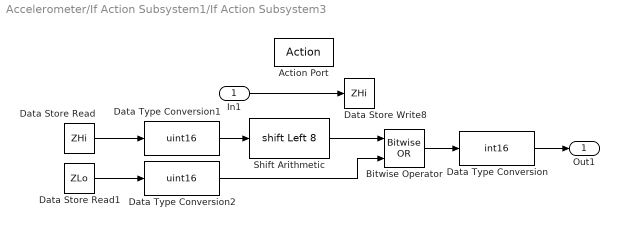
== system Accelerometer/If Action Subsystem1/If Action Subsystem3 ==
  In1 : Inport
  Action Port : ActionPort  ActionPortLabel=if(u1 == 173)
  Bitwise Operator : simulink/Logic and Bit Operations/Bitwise Operator  logicop=OR  UseBitMask=off  NumInputPorts=2  BitMask=bin2dec('11011001')  BitMaskRealWorld=Stored Integer
  Data Store Read : DataStoreRead  DataStoreName=ZHi
  Data Store Read1 : DataStoreRead  DataStoreName=ZLo
  Data Store Write8 : DataStoreWrite  DataStoreName=ZHi
  Data Type Conversion : DataTypeConversion  OutDataTypeStr=int16
  Data Type Conversion1 : DataTypeConversion  OutDataTypeStr=uint16
  Data Type Conversion2 : DataTypeConversion  OutDataTypeStr=uint16
  Shift Arithmetic : ArithShift  BitShiftNumber=8  BitShiftDirection=Left
  Out1 : Outport  VectorParamsAs1DForOutWhenUnconnected=off
  wires:
  In1/1 -> Data Store Write8/1
  Data Store Read1/1 -> Data Type Conversion2/1
  Data Store Read/1 -> Data Type Conversion1/1
  Data Type Conversion/1 -> Out1/1
  Bitwise Operator/1 -> Data Type Conversion/1
  Data Type Conversion2/1 -> Bitwise Operator/2
  Shift Arithmetic/1 -> Bitwise Operator/1
  Data Type Conversion1/1 -> Shift Arithmetic/1

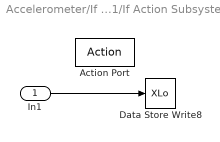
== system Accelerometer/If Action Subsystem1/If Action Subsystem4 ==
  In1 : Inport
  Action Port : ActionPort  ActionPortLabel=if(u1 == 168)
  Data Store Write8 : DataStoreWrite  DataStoreName=XLo
  wires:
  In1/1 -> Data Store Write8/1

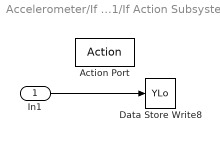
== system Accelerometer/If Action Subsystem1/If Action Subsystem5 ==
  In1 : Inport
  Action Port : ActionPort  ActionPortLabel=if(u1 == 170)
  Data Store Write8 : DataStoreWrite  DataStoreName=YLo
  wires:
  In1/1 -> Data Store Write8/1

== system Accelerometer/If Action Subsystem1/If Action Subsystem6 ==
  In1 : Inport
  Action Port : ActionPort  ActionPortLabel=if(u1 == 172)
  Data Store Write8 : DataStoreWrite  DataStoreName=ZLo
  wires:
  In1/1 -> Data Store Write8/1

== system Accelerometer/If Action Subsystem1/Triggered Subsystem ==
  Trigger : TriggerPort  TriggerType=function-call  VariantControl=Variant
  Constant1 : Constant  OutDataTypeStr=boolean
  Digital_Output1 : mbd_s32k1xx_ec_toolbox/GPIO Blocks/Digital_Output  Priority=1  gpio_pin=PTA11: [PTA11 | Port A I/O]  init_val=High  drive_strength=Low
  wires:
  Constant1/1 -> Digital_Output1/1

== system Accelerometer/Subsystem/Startup Delay ==

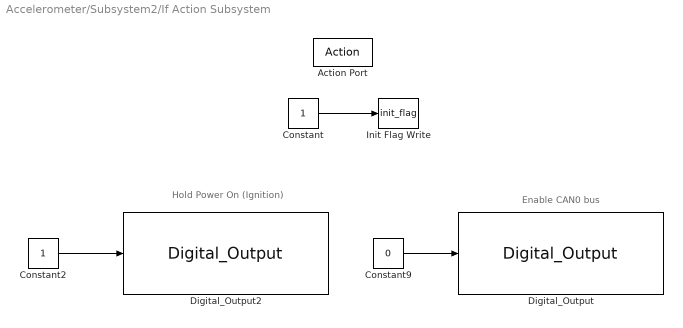
== system Accelerometer/Subsystem2/If Action Subsystem ==
  note: Enable CAN0 bus
  note: Hold Power On (Ignition)
  Action Port : ActionPort  ActionPortLabel=if(u1 == 0)
  Constant : Constant  OutDataTypeStr=uint32
  Constant2 : Constant  OutDataTypeStr=Inherit: Inherit via back propagation
  Constant9 : Constant  Value=0  OutDataTypeStr=Inherit: Inherit via back propagation
  Digital_Output : mbd_s32k1xx_ec_toolbox/GPIO Blocks/Digital_Output  gpio_pin=PTC10: [PTC10 | Port C I/O]  init_val=Low  drive_strength=Low
  Digital_Output2 : mbd_s32k1xx_ec_toolbox/GPIO Blocks/Digital_Output  gpio_pin=PTD7: [PTD7 | Port D I/O]  init_val=High  drive_strength=Low
  Init Flag Write : DataStoreWrite  DataStoreName=init_flag
  wires:
  Constant/1 -> Init Flag Write/1
  Constant9/1 -> Digital_Output/1
  Constant2/1 -> Digital_Output2/1
